simulink model "FourGridNavigation"  (Simulink 7.9)
settings: Solver=ode3  StartTime=0.0  StopTime=4  FixedStep=0.1  RelTol=1e-3
libraries: simulink x1
settings Model: Creator=Karthik Manamcheri  LastModifiedBy=parasara
settings DebuggingCC: FcnCallInpInsideContextMsg=Use local settings
settings GRTTargetCC: CombineOutputUpdateFcns=off  GRTInterface=on

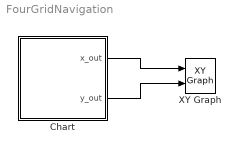
== system FourGridNavigation ==
  Chart : Stateflow chart  TreatAsAtomicUnit=on
  XY Graph : simulink/Sinks/XY Graph  xmin=0  xmax=5  ymin=0  ymax=5  st=-1
  wires:
  Chart/1(x_out) -> XY Graph/1
  Chart/2(y_out) -> XY Graph/2

== stateflow chart Chart ==
  settings: updateMethod=CONTINUOUS
  state Zone1
    du:
    x_dot = vx;
    y_dot = vy;
    vx_dot = -1.2*vx+0.1*vy-0.1;
    vy_dot = 0.1*vx-1.2*vy+1.2;
    x_out = x;
    y_out = y;
  state Zone2
    du:
    x_dot = vx;
    y_dot = vy;
    vx_dot = -1.2*vx+0.1*vy-4.8;
    vy_dot = 0.1*vx-1.2*vy+0.4;
    x_out = x;
    y_out = y;
  state Zone3
    du:
    x_dot = vx;
    y_dot = vy;
    vx_dot = -1.2*vx+0.1*vy+2.4;
    vy_dot = 0.1*vx-1.2*vy-0.2;
    x_out = x;
    y_out = y;
  state Zone4
    du:
    x_dot = vx;
    y_dot = vy;
    vx_dot = -1.2*vx+0.1*vy+3.9;
    vy_dot = 0.1*vx-1.2*vy-3.9;
    x_out = x;
    y_out = y;
  note: @annotation-mode=Zone1;
      | k=1.1;
      | gamma=-0.1;
  note: @annotation-mode=Zone3;
      | k=1.1;
      | gamma=-0.1;
  note: @annotation-mode=Zone2;
      | k=1.1;
      | gamma=-0.1;
  note: @annotation-mode=Zone4;
      | k=1.1;
      | gamma=-0.1;
  Zone1 -> Zone2 [order 1] : [x >= 1 && vx > 0]
  Zone2 -> Zone1 [order 1] : [x <= 1 && vx < 0]
  Zone2 -> Zone4 [order 2] : [y >= 1 && vy > 0]
  Zone4 -> Zone2 [order 1] : [y <= 1 && vy < 0 ]
  Zone1 -> Zone3 [order 2] : [y >= 1 && vy > 0]
  Zone3 -> Zone1 [order 1] : [y <= 1 && vy < 0]
  Zone3 -> Zone4 [order 2] : [x >= 1 && vx > 0]
  Zone4 -> Zone3 [order 2] : [x <= 1 && vx < 0]
  (default) -> Zone1 : {x=0.5; y=0.5;}
  data: x local double; y local double; x_out output double; y_out output double; vx local double; vy local double
  data x settings: updateMethod=SF_CONTINUOUS_TIME_DATA
  data y settings: updateMethod=SF_CONTINUOUS_TIME_DATA
  data vx settings: updateMethod=SF_CONTINUOUS_TIME_DATA
  data vy settings: updateMethod=SF_CONTINUOUS_TIME_DATA
